simulink model "lab3_sim_2k18"  (R2018b)
settings: Solver=FixedStepAuto  StartTime=0.0  StopTime=50  FixedStep=1e-4  RelTol=1e-3
values from neighbouring files (symbols this model uses):
  A = [0, 1, 0, 0;-ks/ms, -T/ms, ks/ms, 0;0, 0, 0, 1;ks/mp, T/mp, -(ks + kp)/mp, -cp/mp]    [lab3_Task_4.m]    (also in lab3_Task_5.m = [0, 1, 0, 0; lab3_Task_5_old.m = [0, 1, 0, 0)
  Ash = [0, 1, 0, 0 ... (first row only)    [getUpdatedModel.m]    (also in lab3_Task_5.m = [0, 0, 0, 0; lab3_Task_5_old.m = [0, 0, 0, 0; lab_3_model_uncertainity.m)
  B = [0, 0; 0, 0; 0, 0; kp/mp, cp/mp]    [lab3_Task_4.m]    (also in lab3_Task_5.m = [0,0,0,0; lab3_Task_5_old.m = [0,0,0,0)
  Bsh = [0,0,0,0 ... (first row only)    [getUpdatedModel.m]    (also in lab3_Task_5.m = [0,0,-1/cz,-1/cz; lab3_Task_5_old.m = [0,0,-1/cz,-1/cz; lab_3_model_uncertainity.m)
  C = [1, 0, 0, 0]    [lab3_Task_4.m]    (also in lab3_Task_5.m = [1, 0, 0, 0; lab3_Task_5_old.m = [1, 0, 0, 0)
  Csh = [1,0, 0, 0 ... (first row only)    [lab3_Task_5.m]    (also in lab3_Task_5_old.m; lab_3_model_uncertainity.m)
  D = 0    [lab3_Task_4.m]    (also in lab3_Task_5.m = zeros(2,4); lab3_Task_5_old.m = zeros(2,4))
  Dsh = zeros(4,4)    [lab3_Task_5.m]    (also in lab3_Task_5_old.m; lab_3_model_uncertainity.m)
  fb_tf = [0, -cz*l2/(l1+l2),0, -cx/(l1+l2) ... (first row only)    [lab3_Task_5.m]    (also in lab3_Task_5_old.m; lab_3_model_uncertainity.m = [0, cz*l2/(l1+l2),0, -cx/(l1+l2))
undefined symbols (not defined in the file or in its folder): sigbuilder_block
settings Model: Creator=Hp  LastModifiedBy=Hp
settings DataIOCC: ReturnWorkspaceOutputs=on

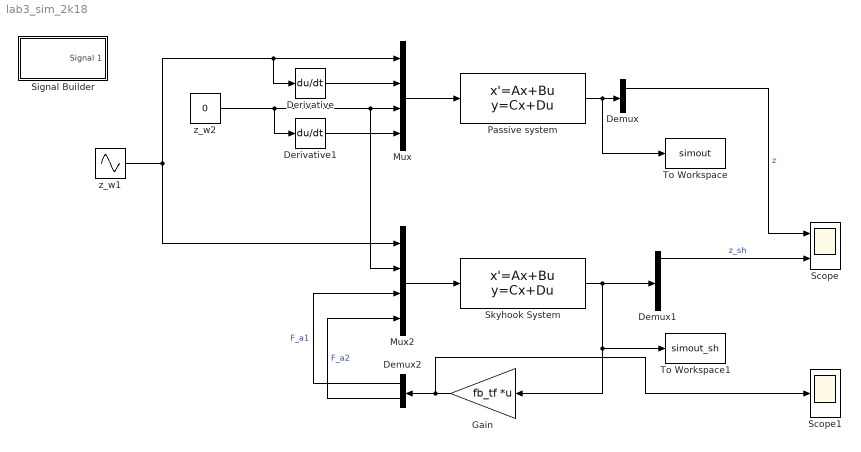
== system lab3_sim_2k18 ==
  Demux : Demux  Outputs=2
  Demux1 : Demux
  Demux2 : Demux  Outputs=2
  Derivative : Derivative
  Derivative1 : Derivative
  Gain : Gain  Gain=fb_tf  Multiplication=Matrix(K*u)
  Mux : Mux
  Mux2 : Mux
  Passive system : StateSpace  A=A  B=B  C=C  D=D  InitialCondition=0  ContinuousStateAttributes={'zs','zs_dot','chi','chi_dot'}
  Scope : Scope  NumInputPorts=2
  Scope1 : Scope
  Signal Builder : Subsystem  Tag=STV Subsys  LoadFcn=sigbuilder_block('load');  StartFcn=sigbuilder_block('start');  StopFcn=sigbuilder_block('stop');  ClipboardFcn=sigbuilder_block('clipboard');  mask(Sigbuilder block){tuvar=[0:10]}
      mask help: Simulink:masks:SigbuilderBlock_MD
      mask init:
      | if ~strcmp(get_param(bdroot(gcbh),'SimulationStatus'),'stopped') tuvar = sigbuilder_block('maskInit'); end
      settings: CopyFcn=sigbuilder_block('copy');  DeleteFcn=sigbuilder_block('delete');  ModelCloseFcn=sigbuilder_block('modelClose');  PreSaveFcn=sigbuilder_block('preSave');  PauseFcn=sigbuilder_block('pause');  ContinueFcn=sigbuilder_block('continue');  NameChangeFcn=sigbuilder_block('namechange');  OpenFcn=sigbuilder_block('open',[5.4 5.5 949.1 474.5 ]);  CloseFcn=sigbuilder_block('close');
      mask Display: plot(0, 0, 100, 100,[2, 2, 32, 32, 2], [68, 8, 8, 68, 68],[32, 2], [38, 38], [32, 19, 2],[53, 60, 44], [32, 17, 17, 2],[16, 16, 31, 31]);txt = getActiveGroup(gcbh);text(2, 100, txt,'verticalAlignment', 'top');
  Skyhook System : StateSpace  A=Ash  B=Bsh  C=Csh  D=Dsh  InitialCondition=0  ContinuousStateAttributes={'zs','zs_dot','chi','chi_dot'}
  To Workspace : ToWorkspace  VariableName=simout  SaveFormat=Timeseries  SampleTime=-1
  To Workspace1 : ToWorkspace  VariableName=simout_sh  SaveFormat=Timeseries  SampleTime=-1
  z_w1 : Sin  Amplitude=0.01  Frequency=6.28  SampleTime=0
  z_w2 : Constant  Value=0
  wires:
  Derivative/1 -> Mux/2
  Mux/1 -> Passive system/1
  z_w2/1 -> Derivative1/1, Mux2/2, Mux/3
  Derivative1/1 -> Mux/4
  Passive system/1 -> To Workspace/1, Demux/1
  Skyhook System/1 -> Gain/1, To Workspace1/1, Demux1/1
  Mux2/1 -> Skyhook System/1
  Demux2/2 -> Mux2/4  "F_a2"
  Demux2/1 -> Mux2/3  "F_a1"
  Gain/1 -> Scope1/1, Demux2/1
  Demux/1 -> Scope/1  "z"
  z_w1/1 -> Derivative/1, Mux/1, Mux2/1
  Demux1/1 -> Scope/2  "z_sh"

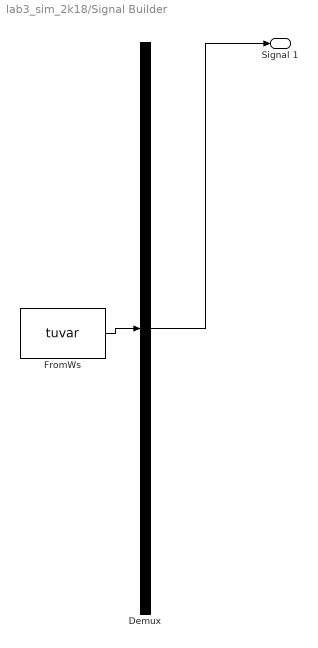
== system lab3_sim_2k18/Signal Builder ==
  Demux : Demux  Tag=STV Demux  Outputs=1
  FromWs : FromWorkspace  Tag=STV FromWs  VariableName=tuvar  SampleTime=0
      SigBuilderData=|
      | common.afterFinalStr = 'Extrapolate'
      | common.sampleTime = 0
      | dataSet.timeRange = [0 60]
      | dataSet.name = 'Group 1'
      | sbobj.Groups.Name = 'Group 1'
      | sbobj.Groups.Signals.Name = 'Signal 1'
      | sbobj.Groups.Signals.XData = [0 33.3 33.3 60]
      | sbobj.Groups.Signals.YData = [0.03 0.03 0 0]
      | sbobj.Groups.TimeRange = [0 60]
  Signal 1 : Outport  Tag=STV Outport
  wires:
  Demux/1 -> Signal 1/1
  FromWs/1 -> Demux/1
